simulink model "two_link_assembly"  (R2024b)
settings: Solver=VariableStepAuto  StartTime=0.0  StopTime=10  RelTol=1e-3
model workspace: external: MATLAB File /Users/mariascarpa/Library/CloudStorage/OneDrive-ImperialCollegeLondon/simulink multibody/two_link_assembly_DataFile.m (data not in the file)
undefined symbols (not defined in the file or in its folder): smiData, X, Y, Z
libraries: sm_lib x17, nesl_utility x7
settings Model: Creator=mariascarpa  LastModifiedBy=mariascarpa

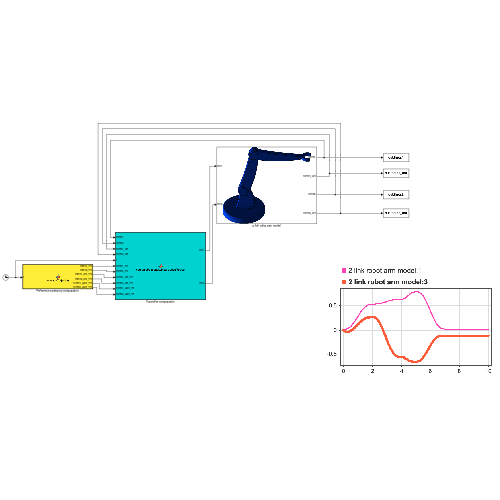
[thumbnail: Simulink's stored preview of the top-level diagram]
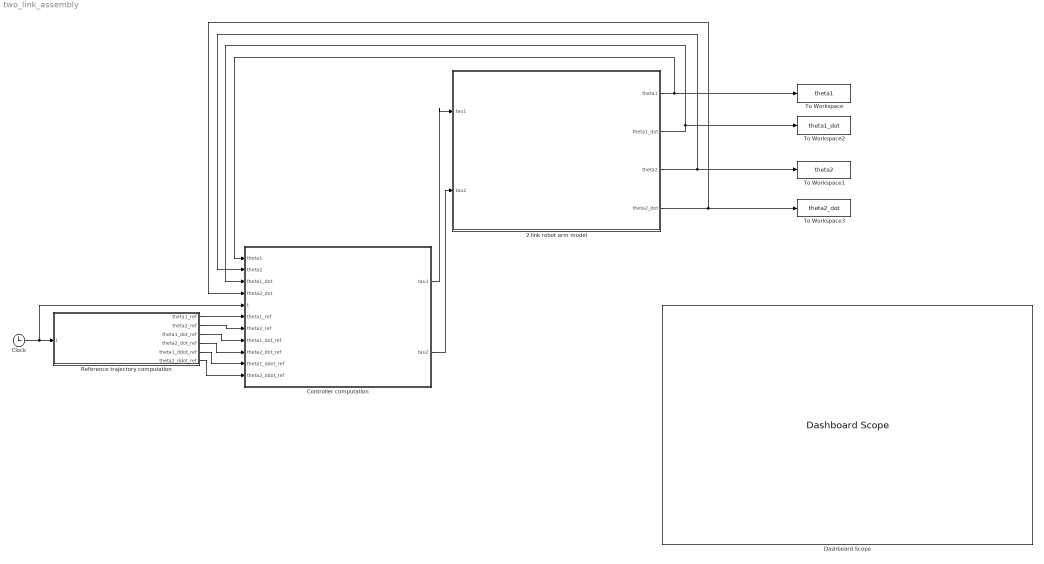
== system two_link_assembly ==
  2 link robot arm model : Subsystem
      mask Display: image('2link_arm.png');
  Clock : Clock
  Controller computation : MATLAB Function  TreatAsAtomicUnit=on
  Dashboard Scope : DashboardScope
  Reference trajectory computation : MATLAB Function  TreatAsAtomicUnit=on
  To Workspace : ToWorkspace  VariableName=theta1  SampleTime=-1
      settings: Save2DSignal=2-D array (concatenate along first dimension)
  To Workspace1 : ToWorkspace  VariableName=theta2  SampleTime=-1
      settings: Save2DSignal=2-D array (concatenate along first dimension)
  To Workspace2 : ToWorkspace  VariableName=theta1_dot  SampleTime=-1
      settings: Save2DSignal=2-D array (concatenate along first dimension)
  To Workspace3 : ToWorkspace  VariableName=theta2_dot  SampleTime=-1
      settings: Save2DSignal=2-D array (concatenate along first dimension)
  wires:
  2 link robot arm model/4(theta2_dot) -> To Workspace3/1, Controller computation/4(theta2_dot)
  2 link robot arm model/3(theta2) -> To Workspace1/1, Controller computation/2(theta2)
  2 link robot arm model/2(theta1_dot) -> To Workspace2/1, Controller computation/3(theta1_dot)
  Reference trajectory computation/1(theta1_ref) -> Controller computation/6(theta1_ref)
  Controller computation/2(tau2) -> 2 link robot arm model/2(tau2)
  Reference trajectory computation/2(theta2_ref) -> Controller computation/7(theta2_ref)
  2 link robot arm model/1(theta1) -> To Workspace/1, Controller computation/1(theta1)
  Reference trajectory computation/4(theta2_dot_ref) -> Controller computation/9(theta2_dot_ref)
  Controller computation/1(tau1) -> 2 link robot arm model/1(tau1)
  Reference trajectory computation/6(theta2_ddot_ref) -> Controller computation/11(theta2_ddot_ref)
  Reference trajectory computation/5(theta1_ddot_ref) -> Controller computation/10(theta1_ddot_ref)
  Reference trajectory computation/3(theta1_dot_ref) -> Controller computation/8(theta1_dot_ref)
  Clock/1 -> Reference trajectory computation/1(t), Controller computation/5(t)

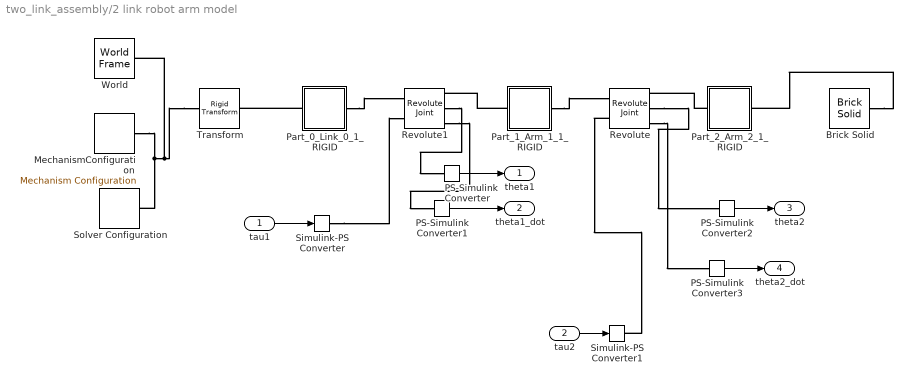
== system two_link_assembly/2 link robot arm model ==
  tau1 : Inport
  tau2 : Inport  Port=2
  Brick Solid : sm_lib/Body Elements/Brick Solid  BrickDimensions=[0.02 0.02 0.1]  BrickDimensionsUnits=m  ExportEntireGeometry=off  InertiaType=CalculateFromGeometry  BasedOnType=Mass  Density=1000  DensityUnits=kg/m^3  Mass=0.01  MassUnits=kg  CenterOfMass=[0 0 0]  CenterOfMassUnits=m  MomentsOfInertia=[1 1 1]  MomentsOfInertiaUnits=kg*m^2  ProductsOfInertia=[0 0 0]  ProductsOfInertiaUnits=kg*m^2  GraphicType=FromGeometry  MarkerShape=Sphere  MarkerSize=10  GraphicVisPropType=AdvancedVisualProperties  GraphicDiffuseColor=[1 0 0]  GraphicOpacity=1  GraphicSpecularColor=[0.5 0.5 0.5 1.0]  GraphicAmbientColor=[0.15 0.15 0.15 1.0]  GraphicEmissiveColor=[0.0 0.0 0.0 1.0]  GraphicShininess=75  DoExposeReferenceFrame=on  SerializedFrames=<Frames/>
  MechanismConfiguration : sm_lib/Utilities/Mechanism Configuration  UniformGravity=Constant  GravityVector=[0 -9.80665 0]  GravityVectorUnits=m/s^2  LinearizationDelta=0.001  JointModeTransitionNonlinearIterations=2
  PS-Simulink Converter{,1..3} (4 alike) : nesl_utility/PS-Simulink Converter  PhysicalDomain=network_engine_domain  SubClassName=ps_output  LeftPortType=input  RightPortType=output  PseudoPeriodic=off  Frequencies=[]  VectorFormat=inherit  Unit=inherit  AffineConversion=off
  Part_0_Link_0_1_RIGID : Subsystem
  Part_1_Arm_1_1_RIGID : Subsystem
  Part_2_Arm_2_1_RIGID : Subsystem
  Revolute : sm_lib/Joints/Revolute Joint  JointMode=Normal  CompositeWrenchDir=FollowerOnBase  CompositeWrenchFrame=BaseFrame  SenseConstraintForce=off  SenseConstraintTorque=off  SenseTotalForce=off  SenseTotalTorque=off  PositionTargetSpecify=off  PositionTargetPriority=Low  PositionTargetValue=smiData.RevoluteJoint(1).Rz.Pos  PositionTargetValueUnits=deg  VelocityTargetSpecify=off  VelocityTargetPriority=High  VelocityTargetValue=0  VelocityTargetValueUnits=deg/s  EquilibriumPosition=0  EquilibriumPositionUnits=deg  SpringStiffness=0  SpringStiffnessUnits=N*m/deg  DampingCoefficient=0  DampingCoefficientUnits=N*m/(deg/s)  LowerLimitSpecify=off  LowerLimitBound=-90  LowerLimitBoundUnits=deg  LowerLimitStiffness=1e4  LowerLimitStiffnessUnits=N*m/deg  LowerLimitDamping=10  LowerLimitDampingUnits=N*m/(deg/s)  LowerLimitTransitionRegionWidth=0.1  LowerLimitTransitionRegionWidthUnits=deg  UpperLimitSpecify=off  UpperLimitBound=90  UpperLimitBoundUnits=deg  UpperLimitStiffness=1e4  UpperLimitStiffnessUnits=N*m/deg  UpperLimitDamping=10  UpperLimitDampingUnits=N*m/(deg/s)  UpperLimitTransitionRegionWidth=0.1  UpperLimitTransitionRegionWidthUnits=deg  TorqueActuationMode=InputTorque  MotionActuationMode=ComputedMotion  SensePosition=on  SenseVelocity=on  SenseAcceleration=off  SenseTorqueForce=off  SenseLowerLimitTorqueForce=off  SenseUpperLimitTorqueForce=off
  Revolute1 : sm_lib/Joints/Revolute Joint  JointMode=Normal  CompositeWrenchDir=FollowerOnBase  CompositeWrenchFrame=BaseFrame  SenseConstraintForce=off  SenseConstraintTorque=off  SenseTotalForce=off  SenseTotalTorque=off  PositionTargetSpecify=off  PositionTargetPriority=Low  PositionTargetValue=smiData.RevoluteJoint(2).Rz.Pos  PositionTargetValueUnits=deg  VelocityTargetSpecify=off  VelocityTargetPriority=High  VelocityTargetValue=0  VelocityTargetValueUnits=deg/s  EquilibriumPosition=0  EquilibriumPositionUnits=deg  SpringStiffness=0  SpringStiffnessUnits=N*m/deg  DampingCoefficient=0  DampingCoefficientUnits=N*m/(deg/s)  LowerLimitSpecify=off  LowerLimitBound=-90  LowerLimitBoundUnits=deg  LowerLimitStiffness=1e4  LowerLimitStiffnessUnits=N*m/deg  LowerLimitDamping=10  LowerLimitDampingUnits=N*m/(deg/s)  LowerLimitTransitionRegionWidth=0.1  LowerLimitTransitionRegionWidthUnits=deg  UpperLimitSpecify=off  UpperLimitBound=90  UpperLimitBoundUnits=deg  UpperLimitStiffness=1e4  UpperLimitStiffnessUnits=N*m/deg  UpperLimitDamping=10  UpperLimitDampingUnits=N*m/(deg/s)  UpperLimitTransitionRegionWidth=0.1  UpperLimitTransitionRegionWidthUnits=deg  TorqueActuationMode=InputTorque  MotionActuationMode=ComputedMotion  SensePosition=on  SenseVelocity=on  SenseAcceleration=off  SenseTorqueForce=off  SenseLowerLimitTorqueForce=off  SenseUpperLimitTorqueForce=off
  Simulink-PS Converter : nesl_utility/Simulink-PS Converter  PhysicalDomain=network_engine_domain  SubClassName=ps_input  LeftPortType=input  RightPortType=output  PseudoPeriodic=off  Frequencies=[]  NoiseDistribution=none  NoiseParameters=[]  Unit=1  AffineConversion=off  FilteringAndDerivatives=provide  SimscapeFilterOrder=1  InputFilterTimeConstant=0.001  UdotUserProvided=0
  Simulink-PS Converter1 : nesl_utility/Simulink-PS Converter  PhysicalDomain=network_engine_domain  SubClassName=ps_input  LeftPortType=input  RightPortType=output  PseudoPeriodic=off  Frequencies=[]  NoiseDistribution=none  NoiseParameters=[]  Unit=1  AffineConversion=off  FilteringAndDerivatives=provide  SimscapeFilterOrder=1  InputFilterTimeConstant=0.001  UdotUserProvided=0
  Solver Configuration : nesl_utility/Solver Configuration  PhysicalDomain=network_engine_domain  SubClassName=solver  LeftPortType=input  RightPortType=generic  Tones=[]  Harmonics=[]  SimulateNoise=off  Profile=off  UseLocalSampling=off  EnableSwitchedLinearOptims=on  FrequencyDomain=off  UseCCode=off  RelTol=0.001  AbsTol=0.001  MinStep=1e-09  ToWorkspace=off  RevertToSquareIcSolve=off  NumHomotopyIterations=100  PhasorMode=off  PhasorModeNumHarmonics=1  ConsistencySolver=NEWTON_XTOL_AFTER_FTOL  IndexReductionMethod=DerivativeReplacement  DoDC=off  ResidualTolerance=1e-09  ConsistencyTolSource=GLOBAL  ConsistencyAbsTol=0.001  ConsistencyRelTol=0.001  ConsistencyTolFactor=0.001  UseLocalSolver=off  LocalSolverChoice=NE_BACKWARD_EULER_ADVANCER  ResolveIndetEquations=on  FunctionEvalNumThread=1  LocalSolverSampleTime=0.001  DoFixedCost=off  MaxNonlinIter=3  MaxModeIter=2  ComputeImpulses=off  ImpulseIterations=2  LinearAlgebra=auto  LinearAlgebraNumThread=0  EquationFormulation=NE_TIME_EF  DelaysMemoryBudget=1024  AutomaticFiltering=on  FilteringTimeConstant=0.001  PartitionStorageMethod=AS_NEEDED  PartitionMemoryBudget=1024  PartitionMethod=ROBUST  MultibodyUseLocalSolver=off  MultibodyLocalSolverChoice=ODE1  MultibodyLocalSolverSampleTime=0.001
  Transform : sm_lib/Frames and Transforms/Rigid Transform  RotationMethod=ArbitraryAxis  FollAlignAxisA=+X  BaseAlignAxisA=+Y  FollAlignAxisB=+Y  BaseAlignAxisB=+Z  RotationStandardAxis=+Z  RotationAngle=smiData.RigidTransform(5).angle  RotationAngleUnits=rad  RotationArbitraryAxis=smiData.RigidTransform(5).axis  RotationSequenceAxes=FollowerAxes  RotationSequence=XYX  RotationSequenceAngles=[0 0 0]  RotationSequenceAnglesUnits=deg  RotationMatrix=[1 0 0;0 1 0;0 0 1]  Quaternion=[1 0 0 0]  TranslationMethod=Cartesian  TranslationCartesianOffset=smiData.RigidTransform(5).translation  TranslationCartesianOffsetUnits=in  TranslationStandardAxis=+Z  TranslationStandardOffset=0  TranslationStandardOffsetUnits=m  TranslationROffset=0  TranslationROffsetUnits=m  TranslationThetaOffset=0  TranslationThetaOffsetUnits=deg  TranslationZOffset=0  TranslationZOffsetUnits=m
  World : sm_lib/Frames and Transforms/World Frame
  theta1 : Outport
  theta1_dot : Outport  Port=2
  theta2 : Outport  Port=3
  theta2_dot : Outport  Port=4
  wires:
  PS-Simulink Converter2/1 -> theta2/1
  tau1/1 -> Simulink-PS Converter/1
  PS-Simulink Converter1/1 -> theta1_dot/1
  tau2/1 -> Simulink-PS Converter1/1
  PS-Simulink Converter3/1 -> theta2_dot/1
  PS-Simulink Converter/1 -> theta1/1
  connections:
  Revolute/RConn3 -- PS-Simulink Converter3/LConn1
  Part_0_Link_0_1_RIGID/RConn1 -- Revolute1/LConn1
  Part_2_Arm_2_1_RIGID/LConn1 -- Revolute/RConn1
  Revolute/RConn2 -- PS-Simulink Converter2/LConn1
  Simulink-PS Converter/RConn1 -- Revolute1/LConn2
  Transform/LConn1 -- MechanismConfiguration/RConn1 -- Solver Configuration/RConn1 -- World/RConn1
  Revolute/LConn2 -- Simulink-PS Converter1/RConn1
  Part_1_Arm_1_1_RIGID/RConn1 -- Revolute/LConn1
  Revolute1/RConn2 -- PS-Simulink Converter/LConn1
  Revolute1/RConn3 -- PS-Simulink Converter1/LConn1
  Part_1_Arm_1_1_RIGID/LConn1 -- Revolute1/RConn1
  Part_0_Link_0_1_RIGID/LConn1 -- Transform/RConn1
  Brick Solid/RConn1 -- Part_2_Arm_2_1_RIGID/RConn1

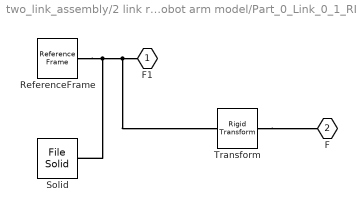
== system two_link_assembly/2 link robot arm model/Part_0_Link_0_1_RIGID ==
  ReferenceFrame : sm_lib/Frames and Transforms/Reference Frame
  Solid : sm_lib/Body Elements/File Solid  ExtGeomFileName=Part_0_Link__0_Varsayilan_sldprt.STEP  UnitType=FromFile  ExtGeomFileUnits=m  StepReaderType=HEX  ExportConvexHullGeometry=off  InertiaType=Custom  BasedOnType=DensityFromFile  Density=1000  DensityUnits=kg/m^3  Mass=smiData.Solid(3).mass  MassUnits=kg  CenterOfMass=smiData.Solid(3).CoM  CenterOfMassUnits=mm  MomentsOfInertia=smiData.Solid(3).MoI  MomentsOfInertiaUnits=kg*mm^2  ProductsOfInertia=smiData.Solid(3).PoI  ProductsOfInertiaUnits=kg*mm^2  GraphicType=FromGeometry  MarkerShape=Sphere  MarkerSize=10  GraphicVisPropType=SimpleVisualProperties  GraphicDiffuseColor=smiData.Solid(3).color  GraphicOpacity=smiData.Solid(3).opacity  GraphicSpecularColor=[0.5 0.5 0.5 1.0]  GraphicAmbientColor=[0.15 0.15 0.15 1.0]  GraphicEmissiveColor=[0.0 0.0 0.0 1.0]  GraphicShininess=75  DoExposeReferenceFrame=on  SerializedFrames=<Frames/>
  Transform : sm_lib/Frames and Transforms/Rigid Transform  RotationMethod=ArbitraryAxis  FollAlignAxisA=+X  BaseAlignAxisA=+Y  FollAlignAxisB=+Y  BaseAlignAxisB=+Z  RotationStandardAxis=+Z  RotationAngle=smiData.RigidTransform(3).angle  RotationAngleUnits=rad  RotationArbitraryAxis=smiData.RigidTransform(3).axis  RotationSequenceAxes=FollowerAxes  RotationSequence=XYX  RotationSequenceAngles=[0 0 0]  RotationSequenceAnglesUnits=deg  RotationMatrix=[1 0 0;0 1 0;0 0 1]  Quaternion=[1 0 0 0]  TranslationMethod=Cartesian  TranslationCartesianOffset=smiData.RigidTransform(3).translation  TranslationCartesianOffsetUnits=in  TranslationStandardAxis=+Z  TranslationStandardOffset=0  TranslationStandardOffsetUnits=m  TranslationROffset=0  TranslationROffsetUnits=m  TranslationThetaOffset=0  TranslationThetaOffsetUnits=deg  TranslationZOffset=0  TranslationZOffsetUnits=m
  F1 : PMIOPort  Side=Left
  F : PMIOPort  Port=2  Side=Right
  connections:
  Solid/RConn1 -- ReferenceFrame/RConn1 -- Transform/LConn1 -- F1/RConn1
  Transform/RConn1 -- F/RConn1

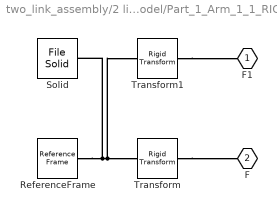
== system two_link_assembly/2 link robot arm model/Part_1_Arm_1_1_RIGID ==
  ReferenceFrame : sm_lib/Frames and Transforms/Reference Frame
  Solid : sm_lib/Body Elements/File Solid  ExtGeomFileName=Part_1_Arm__1_Varsayilan_sldprt.STEP  UnitType=FromFile  ExtGeomFileUnits=m  StepReaderType=HEX  ExportConvexHullGeometry=off  InertiaType=Custom  BasedOnType=DensityFromFile  Density=1000  DensityUnits=kg/m^3  Mass=smiData.Solid(2).mass  MassUnits=kg  CenterOfMass=smiData.Solid(2).CoM  CenterOfMassUnits=mm  MomentsOfInertia=smiData.Solid(2).MoI  MomentsOfInertiaUnits=kg*mm^2  ProductsOfInertia=smiData.Solid(2).PoI  ProductsOfInertiaUnits=kg*mm^2  GraphicType=FromGeometry  MarkerShape=Sphere  MarkerSize=10  GraphicVisPropType=SimpleVisualProperties  GraphicDiffuseColor=smiData.Solid(2).color  GraphicOpacity=smiData.Solid(2).opacity  GraphicSpecularColor=[0.5 0.5 0.5 1.0]  GraphicAmbientColor=[0.15 0.15 0.15 1.0]  GraphicEmissiveColor=[0.0 0.0 0.0 1.0]  GraphicShininess=75  DoExposeReferenceFrame=on  SerializedFrames=<Frames/>
  Transform : sm_lib/Frames and Transforms/Rigid Transform  RotationMethod=ArbitraryAxis  FollAlignAxisA=+X  BaseAlignAxisA=+Y  FollAlignAxisB=+Y  BaseAlignAxisB=+Z  RotationStandardAxis=+Z  RotationAngle=smiData.RigidTransform(1).angle  RotationAngleUnits=rad  RotationArbitraryAxis=smiData.RigidTransform(1).axis  RotationSequenceAxes=FollowerAxes  RotationSequence=XYX  RotationSequenceAngles=[0 0 0]  RotationSequenceAnglesUnits=deg  RotationMatrix=[1 0 0;0 1 0;0 0 1]  Quaternion=[1 0 0 0]  TranslationMethod=Cartesian  TranslationCartesianOffset=smiData.RigidTransform(1).translation  TranslationCartesianOffsetUnits=in  TranslationStandardAxis=+Z  TranslationStandardOffset=0  TranslationStandardOffsetUnits=m  TranslationROffset=0  TranslationROffsetUnits=m  TranslationThetaOffset=0  TranslationThetaOffsetUnits=deg  TranslationZOffset=0  TranslationZOffsetUnits=m
  Transform1 : sm_lib/Frames and Transforms/Rigid Transform  RotationMethod=ArbitraryAxis  FollAlignAxisA=+X  BaseAlignAxisA=+Y  FollAlignAxisB=+Y  BaseAlignAxisB=+Z  RotationStandardAxis=+Z  RotationAngle=smiData.RigidTransform(4).angle  RotationAngleUnits=rad  RotationArbitraryAxis=smiData.RigidTransform(4).axis  RotationSequenceAxes=FollowerAxes  RotationSequence=XYX  RotationSequenceAngles=[0 0 0]  RotationSequenceAnglesUnits=deg  RotationMatrix=[1 0 0;0 1 0;0 0 1]  Quaternion=[1 0 0 0]  TranslationMethod=Cartesian  TranslationCartesianOffset=smiData.RigidTransform(4).translation  TranslationCartesianOffsetUnits=in  TranslationStandardAxis=+Z  TranslationStandardOffset=0  TranslationStandardOffsetUnits=m  TranslationROffset=0  TranslationROffsetUnits=m  TranslationThetaOffset=0  TranslationThetaOffsetUnits=deg  TranslationZOffset=0  TranslationZOffsetUnits=m
  F1 : PMIOPort  Side=Left
  F : PMIOPort  Port=2  Side=Right
  connections:
  Solid/RConn1 -- ReferenceFrame/RConn1 -- Transform/LConn1 -- Transform1/LConn1
  Transform/RConn1 -- F/RConn1
  Transform1/RConn1 -- F1/RConn1

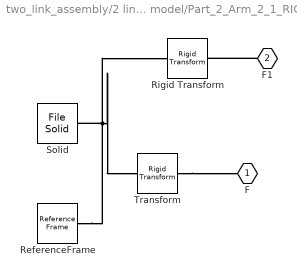
== system two_link_assembly/2 link robot arm model/Part_2_Arm_2_1_RIGID ==
  ReferenceFrame : sm_lib/Frames and Transforms/Reference Frame
  Rigid Transform : sm_lib/Frames and Transforms/Rigid Transform  RotationMethod=StandardAxis  FollAlignAxisA=+X  BaseAlignAxisA=+Y  FollAlignAxisB=+Y  BaseAlignAxisB=+Z  RotationStandardAxis=+X  RotationAngle=90  RotationAngleUnits=deg  RotationArbitraryAxis=[0 0 1]  RotationSequenceAxes=FollowerAxes  RotationSequence=XYX  RotationSequenceAngles=[0 0 0]  RotationSequenceAnglesUnits=deg  RotationMatrix=[1 0 0;0 1 0;0 0 1]  Quaternion=[1 0 0 0]  TranslationMethod=Cartesian  TranslationCartesianOffset=[0.1 0 0]  TranslationCartesianOffsetUnits=m  TranslationStandardAxis=+Z  TranslationStandardOffset=0  TranslationStandardOffsetUnits=m  TranslationROffset=0  TranslationROffsetUnits=m  TranslationThetaOffset=0  TranslationThetaOffsetUnits=deg  TranslationZOffset=0  TranslationZOffsetUnits=m
  Solid : sm_lib/Body Elements/File Solid  ExtGeomFileName=Part_2_Arm__2_Varsayilan_sldprt.STEP  UnitType=FromFile  ExtGeomFileUnits=m  StepReaderType=HEX  ExportConvexHullGeometry=off  InertiaType=Custom  BasedOnType=DensityFromFile  Density=1000  DensityUnits=kg/m^3  Mass=smiData.Solid(1).mass  MassUnits=kg  CenterOfMass=smiData.Solid(1).CoM  CenterOfMassUnits=mm  MomentsOfInertia=smiData.Solid(1).MoI  MomentsOfInertiaUnits=kg*mm^2  ProductsOfInertia=smiData.Solid(1).PoI  ProductsOfInertiaUnits=kg*mm^2  GraphicType=FromGeometry  MarkerShape=Sphere  MarkerSize=10  GraphicVisPropType=SimpleVisualProperties  GraphicDiffuseColor=smiData.Solid(1).color  GraphicOpacity=smiData.Solid(1).opacity  GraphicSpecularColor=[0.5 0.5 0.5 1.0]  GraphicAmbientColor=[0.15 0.15 0.15 1.0]  GraphicEmissiveColor=[0.0 0.0 0.0 1.0]  GraphicShininess=75  DoExposeReferenceFrame=on  SerializedFrames=<Frames/>
  Transform : sm_lib/Frames and Transforms/Rigid Transform  RotationMethod=ArbitraryAxis  FollAlignAxisA=+X  BaseAlignAxisA=+Y  FollAlignAxisB=+Y  BaseAlignAxisB=+Z  RotationStandardAxis=+Z  RotationAngle=smiData.RigidTransform(2).angle  RotationAngleUnits=rad  RotationArbitraryAxis=smiData.RigidTransform(2).axis  RotationSequenceAxes=FollowerAxes  RotationSequence=XYX  RotationSequenceAngles=[0 0 0]  RotationSequenceAnglesUnits=deg  RotationMatrix=[1 0 0;0 1 0;0 0 1]  Quaternion=[1 0 0 0]  TranslationMethod=Cartesian  TranslationCartesianOffset=smiData.RigidTransform(2).translation  TranslationCartesianOffsetUnits=in  TranslationStandardAxis=+Z  TranslationStandardOffset=0  TranslationStandardOffsetUnits=m  TranslationROffset=0  TranslationROffsetUnits=m  TranslationThetaOffset=0  TranslationThetaOffsetUnits=deg  TranslationZOffset=0  TranslationZOffsetUnits=m
  F : PMIOPort  Side=Left
  F1 : PMIOPort  Port=2  Side=Right
  connections:
  ReferenceFrame/RConn1 -- Transform/LConn1 -- Rigid Transform/LConn1 -- Solid/RConn1
  Transform/RConn1 -- F/RConn1
  F1/RConn1 -- Rigid Transform/RConn1

== matlab function two_link_assembly/Reference trajectory computation ==
  data: t input; theta1_ref output; theta2_ref output; theta1_dot_ref output; theta2_dot_ref output; theta1_ddot_ref output; theta2_ddot_ref output
function [theta1_ref, theta2_ref, theta1_dot_ref, theta2_dot_ref, theta1_ddot_ref, theta2_ddot_ref] = generateTrajectory(t)
% Inputs:
    %   t - Current time (seconds)

% Outputs:
    %   theta1_ref, theta2_ref - Joint angle references (rad)
    %   theta1_dot_ref, theta2_dot_ref - Joint velocity references (rad/s)
    %   theta1_ddot_ref, theta2_ddot_ref - Joint acceleration references (rad/s²)
        L1 = 1;
        L2 = 1;
        if t < 3
                % Move to pickup location using smooth trajectory
                [theta1_ref, theta2_ref, theta1_dot_ref, theta2_dot_ref, theta1_ddot_ref, theta2_ddot_ref] = ...
                    smoothTrajectory(t, 0, 3, 0, pi/6, 0, -pi/4, L1, L2);
                
            elseif t < 4
                % Hold at pickup (grasping)
                theta1_ref = pi/6;
                theta2_ref = -pi/4;
                theta1_dot_ref = 0;
                theta2_dot_ref = 0;
                theta1_ddot_ref = 0;
                theta2_ddot_ref = 0;
                
            elseif t < 8
                % Transport to dropoff location
                [theta1_ref, theta2_ref, theta1_dot_ref, theta2_dot_ref, theta1_ddot_ref, theta2_ddot_ref] = ...
                    smoothTrajectory(t-4, 0, 4, pi/6, -pi/6, -pi/4, pi/3, L1, L2);
                
            elseif t < 9
                % Hold at dropoff (releasing)
                theta1_ref = -pi/6;
                theta2_ref = pi/3;
                theta1_dot_ref = 0;
                theta2_dot_ref = 0;
                theta1_ddot_ref = 0;
                theta2_ddot_ref = 0;
                
            else
                % Return to home position
                [theta1_ref, theta2_ref, theta1_dot_ref, theta2_dot_ref, theta1_ddot_ref, theta2_ddot_ref] = ...
                    smoothTrajectory(t-9, 0, 3, -pi/6, 0, pi/3, 0, L1, L2);
          end
  
end



function [theta1, theta2, theta1_dot, theta2_dot, theta1_ddot, theta2_ddot] = ...
    smoothTrajectory(t, t_start, duration, theta1_i, theta1_f, theta2_i, theta2_f, L1, L2)
    % Creates smooth trajectory from initial to final angles using 5th order polynomial
    
    if t < t_start
        theta1 = theta1_i;
        theta2 = theta2_i;
        theta1_dot = 0;
        theta2_dot = 0;
        theta1_ddot = 0;
        theta2_ddot = 0;
    elseif t < t_start + duration
        % Normalized time [0, 1]
        s = (t - t_start) / duration;
        
        % 5th order polynomial 
        sigma = 10*s^3 - 15*s^4 + 6*s^5;
        sigma_dot = (30*s^2 - 60*s^3 + 30*s^4) / duration;
        sigma_ddot = (60*s - 180*s^2 + 120*s^3) / duration^2;
        
        % Interpolate
        theta1 = theta1_i + (theta1_f - theta1_i) * sigma;
        theta2 = theta2_i + (theta2_f - theta2_i) * sigma;
        
        theta1_dot = (theta1_f - theta1_i) * sigma_dot;
        theta2_dot = (theta2_f - theta2_i) * sigma_dot;
        
        theta1_ddot = (theta1_f - theta1_i) * sigma_ddot;
        theta2_ddot = (theta2_f - theta2_i) * sigma_ddot;
    else
        theta1 = theta1_f;
        theta2 = theta2_f;
        theta1_dot = 0;
        theta2_dot = 0;
        theta1_ddot = 0;
        theta2_ddot = 0;
    end
end

== matlab function two_link_assembly/Controller computation ==
  data: theta1 input; tau1 output; theta2 input; theta1_dot input; theta2_dot input; tau2 output; t input; theta1_ref input; theta2_ref input; theta1_dot_ref input; theta2_dot_ref input; theta1_ddot_ref input; theta2_ddot_ref input
function [tau1, tau2] = computeFeedbackLinearizationTorque(theta1, theta2, theta1_dot, theta2_dot,t,theta1_ref,theta2_ref,theta1_dot_ref,theta2_dot_ref,theta1_ddot_ref,theta2_ddot_ref)
    % COMPUTEFEEDBACKlinearizationtorque - Computes control torques using feedback linearization
    %
    % This function implements computed torque control (feedback linearization) for a
    % two-link planar robot arm. It cancels the nonlinear dynamics and allows linear
    % control design on the resulting double integrator system.
    %
    % Inputs:
    %   theta1      - Joint 1 angle (rad)
    %   theta2      - Joint 2 angle (rad)
    %   theta1_dot  - Joint 1 velocity (rad/s)
    %   theta2_dot  - Joint 2 velocity (rad/s)
    %
    % Outputs:
    %   tau1 - Torque for joint 1 (N⋅m)
    %   tau2 - Torque for joint 2 (N⋅m)
    %
    % Theory:
    %   Robot dynamics: M(θ)⋅θ̈ = τ - C(θ,θ̇) - G(θ)
    %   
    %   Control law: τ = M(θ)⋅(θ̈_ref + u) + C(θ,θ̇) + G(θ)
    %   
    %   Result: θ̈ = θ̈_ref + u (linearized dynamics!)
    %

    
    %% System Parameters
    
    M1 = 0.1146727860355552;    % Mass of link 1 (kg)
    M2 = 0.09704921309928316;    % Mass of link 2 (kg)
    L1 = 1;    % Length of link 1 (m)
    L2 = 1;    % Length of link 2 (m)
    g = 0;    % Gravitational acceleration (m/s²)
    
    amp1 = pi/6;
    amp2 = pi/8;
    freq1 = 0.2;
    freq2 = 0.15;


    %% Reference Trajectory (Regulation to origin)
 
    
    % State vector for game controller
    x = [theta1 - theta1_ref;
         theta2 - theta2_ref;
         theta1_dot - theta1_dot_ref;
         theta2_dot - theta2_dot_ref];

    % Game theory parameters
    gamma1 = 15;
    gamma2 = 20;

    % Cost matrices
    Q1 = 0.4 * eye(4);
    Q2 = 0.2 * eye(4);

    % Control weight matrices
    R1 = eye(2) / gamma1;
    R2 = eye(2) / gamma2;

    % Solved Riccati equations and game theory controllers
    K1 = [50, 0, 8, 0;
          0, 12, 0, 6];

    K2 = [50, 0, 5, 0;
          0, 8, 0, 4];

    % Nash equilibrium control
    u1 = -K1 * x;
    u2 = -K2 * x;
    u_total = u1 + u2;

    % Compute M, C, G (same as before)
    M11 = M1*L1^2 + M2*(L1^2 + L2^2 + 2*L1*L2*cos(theta2));
    M12 = M2*(L2^2 + L1*L2*cos(theta2));
    M22 = M2*L2^2;
    M = [M11, M12; M12, M22];

    h = -M2*L1*L2*sin(theta2);
    C = [h*(2*theta1_dot*theta2_dot + theta2_dot^2); h*theta1_dot^2];

    G = [(M1 + M2)*g*L1*cos(theta1) + M2*g*L2*cos(theta1 + theta2);
         M2*g*L2*cos(theta1 + theta2)];

    % Feedback linearization
    theta_ddot_ref = [theta1_ddot_ref; theta2_ddot_ref];
    tau = M * (theta_ddot_ref + u_total) + C + G;

    tau1 = tau(1);
    tau2 = tau(2);    
end
